simulink model "Coordinate_Systems_2020a"  (R2024b)
settings: Solver=VariableStepAuto  StartTime=0.0  StopTime=1000  RelTol=1e-3
undefined symbols (not defined in the file or in its folder): drawAircraft
libraries: simulink x6
settings Model: Creator=h1huang  LastModifiedBy=Administrator
settings SolverCC: AlgebraicLoopSolver=TrustRegion
settings DebuggingCC: UnconnectedInputMsg=warning  UnconnectedOutputMsg=warning  UnconnectedLineMsg=warning
settings ModelReferenceCC: EnableRefExpFcnMdlSchedulingChecks=on
settings RTWCC: GPUComputeCapability=3.5  DLArmComputeVersion=19.05

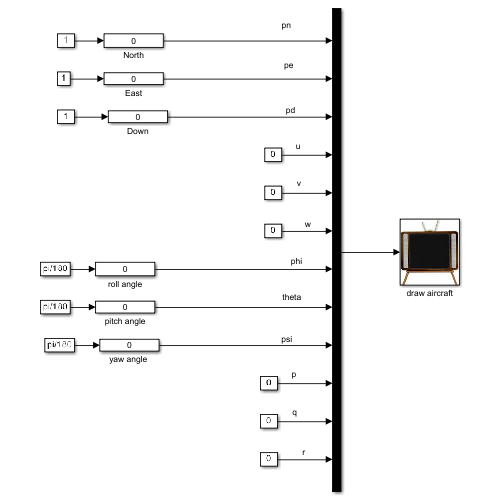
[thumbnail: Simulink's stored preview of the top-level diagram]
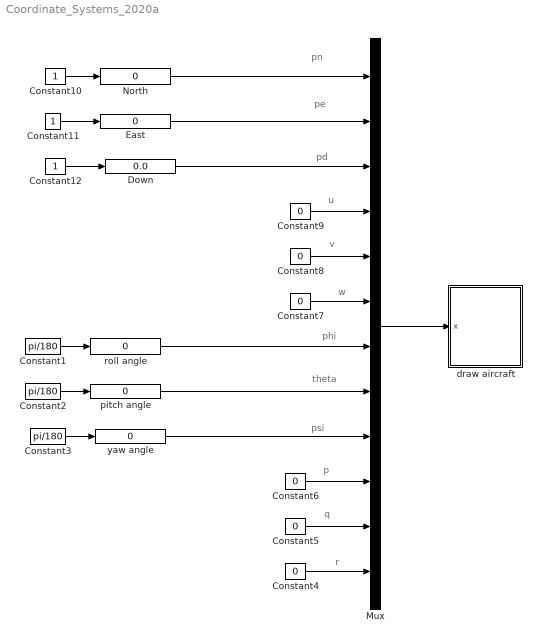
== system Coordinate_Systems_2020a ==
  note: q
  note: r
  note: pe
  note: psi
  note: pd
  note: p
  note: pn
  note: theta
  note: phi
  note: u
  note: v
  note: w
  Constant1 : Constant  Value=pi/180
  Constant10 : Constant
  Constant11 : Constant
  Constant12 : Constant
  Constant2 : Constant  Value=pi/180
  Constant3 : Constant  Value=pi/180
  Constant{4..9} (6 alike) : Constant  Value=0
  Down : simulink/Math Operations/Slider Gain  gain=0.0  low=-1000  high=0
  East : simulink/Math Operations/Slider Gain  gain=0  low=-1000  high=1000
  Mux : Mux  Inputs=12
  North : simulink/Math Operations/Slider Gain  gain=0  low=-900  high=900
  draw aircraft : Subsystem
      mask Display: image(imread('tv.jpg'))
  pitch angle : simulink/Math Operations/Slider Gain  gain=0  low=-180  high=180
  roll angle : simulink/Math Operations/Slider Gain  gain=0  low=-180  high=180
  "yaw angle " : simulink/Math Operations/Slider Gain  gain=0  low=-180  high=180
  wires:
  Constant2/1 -> pitch angle/1
  Constant12/1 -> Down/1
  North/1 -> Mux/1
  Constant8/1 -> Mux/5
  Constant7/1 -> Mux/6
  Constant10/1 -> North/1
  Constant9/1 -> Mux/4
  roll angle/1 -> Mux/7
  Down/1 -> Mux/3
  Constant11/1 -> East/1
  East/1 -> Mux/2
  Constant4/1 -> Mux/12
  Constant6/1 -> Mux/10
  Constant5/1 -> Mux/11
  Constant3/1 -> "yaw angle "/1
  pitch angle/1 -> Mux/8
  Constant1/1 -> roll angle/1
  "yaw angle "/1 -> Mux/9
  Mux/1 -> draw aircraft/1(x)

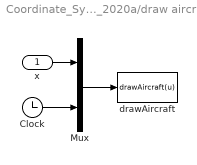
== system Coordinate_Systems_2020a/draw aircraft ==
  x : Inport
  Clock : Clock
  Mux : Mux  Inputs=2
  drawAircraft : MATLABFcn  MATLABFcn=drawAircraft(u)  OutputDimensions=0  SampleTime=0.1
  wires:
  Mux/1 -> drawAircraft/1
  x/1 -> Mux/1
  Clock/1 -> Mux/2
